simulink model "simulink_discrete_3"  (Simulink 7.7)
settings: Solver=ode45  StartTime=0.0  StopTime=0.7  RelTol=1e-3
undefined symbols (not defined in the file or in its folder): T1, T2
libraries: cstblocks x6, simulink x2, dsparch4 x1
settings Model: Creator=Koldo  LastModifiedBy=Koldo

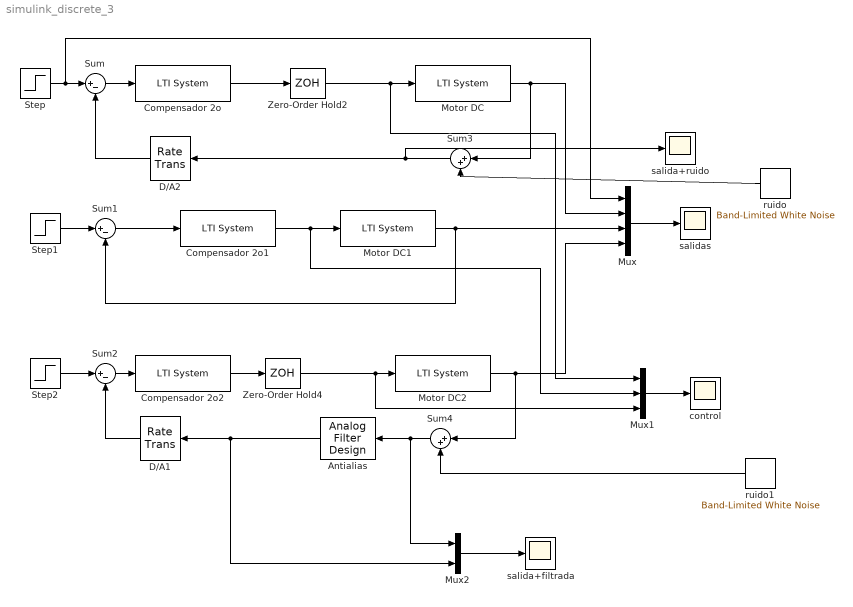
== system simulink_discrete_3 ==
  Antialias : dsparch4/Analog Filter Design  method=Butterworth  filttype=Lowpass  N=5  Wlo=340  Whi=80  Rp=2  Rs=40
  Compensador 2o : cstblocks/LTI System  SystemSampleTime=-1  sys=CT2_tust  IC=[]
  Compensador 2o1 : cstblocks/LTI System  SystemSampleTime=-1  sys=C  IC=[]
  Compensador 2o2 : cstblocks/LTI System  SystemSampleTime=-1  sys=CT1_tust  IC=[]
  D/A1 : RateTransition  Integrity=off  Deterministic=off  X0=8.96  OutPortSampleTime=T1
  D/A2 : RateTransition  Integrity=off  Deterministic=off  X0=8.96  OutPortSampleTime=T2
  Motor DC : cstblocks/LTI System  SystemSampleTime=-1  sys=G  IC=[]
  Motor DC1 : cstblocks/LTI System  SystemSampleTime=-1  sys=G  IC=[]
  Motor DC2 : cstblocks/LTI System  SystemSampleTime=-1  sys=G  IC=[]
  Mux : Mux
  Mux1 : Mux  Inputs=3
  Mux2 : Mux  Inputs=2
  Step : Step  Time=0.1  SampleTime=0
  Step1 : Step  Time=0.1  SampleTime=0
  Step2 : Step  Time=0.1  SampleTime=0
  Sum : Sum  Inputs=|+-
  Sum1 : Sum  Inputs=|+-
  Sum2 : Sum  Inputs=|+-
  Sum3 : Sum  Inputs=|++
  Sum4 : Sum  Inputs=|++
  Zero-Order Hold2 : ZeroOrderHold  SampleTime=T2
  Zero-Order Hold4 : ZeroOrderHold  SampleTime=T1
  control : Scope
      settings: MaxDataPoints=50000
  ruido : simulink/Sources/Band-Limited White Noise  SystemSampleTime=-1  Cov=[0.0000001]  Ts=0.0001  seed=[23341]
  ruido1 : simulink/Sources/Band-Limited White Noise  SystemSampleTime=-1  Cov=[0.0000001]  Ts=0.0001  seed=[23341]
  salida+filtrada : Scope
      settings: SaveName=ScopeData3  MaxDataPoints=50000
  salida+ruido : Scope
      settings: SaveName=ScopeData2  MaxDataPoints=50000
  salidas : Scope
      settings: MaxDataPoints=50000
  wires:
  Step/1 -> Mux/1, Sum/1
  Sum/1 -> Compensador 2o/1
  Motor DC/1 -> Mux/2, Sum3/1
  Compensador 2o/1 -> Zero-Order Hold2/1
  Zero-Order Hold2/1 -> Motor DC/1, Mux1/1
  Step1/1 -> Sum1/1
  Sum1/1 -> Compensador 2o1/1
  Motor DC1/1 -> Mux/3, Sum1/2
  Compensador 2o1/1 -> Motor DC1/1, Mux1/2
  Mux/1 -> salidas/1
  Step2/1 -> Sum2/1
  Sum2/1 -> Compensador 2o2/1
  Motor DC2/1 -> Mux/4, Sum4/1
  Zero-Order Hold4/1 -> Motor DC2/1, Mux1/3
  Mux1/1 -> control/1
  D/A1/1 -> Sum2/2
  Compensador 2o2/1 -> Zero-Order Hold4/1
  Sum3/1 -> salida+ruido/1, D/A2/1
  ruido/1 -> Sum3/2
  Sum4/1 -> Antialias/1, Mux2/1
  Antialias/1 -> Mux2/2, D/A1/1
  ruido1/1 -> Sum4/2
  Mux2/1 -> salida+filtrada/1
  D/A2/1 -> Sum/2
